simulink model "ECU_Controller"  (R2025b)
settings: Solver=FixedStepAuto  StartTime=0.0  StopTime=10.0  RelTol=1e-3  EnableMultiTasking=on
libraries: stm32f4xxblockslib x2
settings Model: STM32="{\"AnalogInput\":[{\"ID\":\"PIL_System_POTS:37\"},{\"ID\":\"PIL_System_POTS:38\"}]}"  Creator=Lakshay Taneja  LastModifiedBy=Lakshay Taneja
settings OptimizationCC: DefaultParameterBehavior=Inlined  EnhancedBackFolding=on  PassReuseOutputArgsAs=Individual arguments  ZeroExternalMemoryAtStartup=off  ZeroInternalMemoryAtStartup=off  MaxStackSize=512  OptimizeBlockOrder=speed  DifferentSizesBufferReuse=on  OptimizationCustomize=off  EfficientTunableParamExpr=on
settings DebuggingCC: ParameterTunabilityLossMsg=error
settings HardwareCC: ProdBitPerPointer=32.0  ProdBitPerSizeT=32.0  ProdBitPerPtrDiffT=32.0  ProdLargestAtomicInteger=Long  ProdLargestAtomicFloat=Double  ProdWordSize=32.0  ProdLongLongMode=on  ProdHWDeviceType=ARM Compatible->ARM Cortex-M
settings SFSimCC: MATLABDynamicMemAlloc=off
settings RTWCC: SystemTargetFile=ert.tlc  HardwareBoard=STM32F4xx Based  TemplateMakefile=ert_default_tmf  Toolchain=GNU Tools for ARM Embedded Processors  CreateSILPILBlock=PIL  Description=Embedded Coder
settings CodeAppCC: ForceParamTrailComments=on  IgnoreCustomStorageClasses=off  OperatorAnnotations=on  SimulinkDataObjDesc=on  SFDataObjDesc=on  InsertBlockDesc=on
settings ERTTargetCC: ExtModeTransport=3.0  ExtModeStaticAlloc=on  ExtModeStaticAllocSize=2048.0  ExtModeMexFile=ext_xcp  ExtModeIntrfLevel=Level2 - Open  TargetLangStandard=C99 (ISO)  CodeReplacementLibrary=ARM Cortex-M

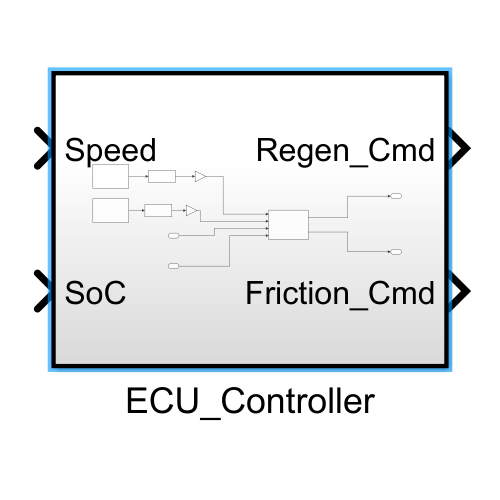
[thumbnail: Simulink's stored preview of the top-level diagram]
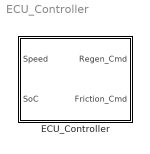
== system ECU_Controller ==
  ECU_Controller : Subsystem  TreatAsAtomicUnit=on

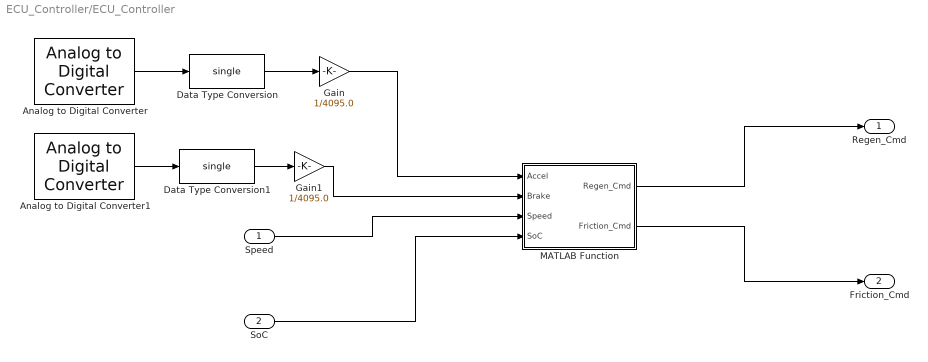
== system ECU_Controller/ECU_Controller ==
  Speed : Inport  OutDataTypeStr=single
  SoC : Inport  Port=2  OutDataTypeStr=single
  Analog to Digital Converter : stm32f4xxblockslib/Analog to Digital Converter  ADCModule=ADC1  ConversionGroup=Regular  TriggerMode=Trigger and read  NumberOfConversions=1  EnableBufferConv=off  BufferLength=1  OutputStatus=off  SampleTime=0.01  EnableSimPort=off  hoistedMaskSrc=ECSoC/ECSimCodegen/Analog to Digital Converter
      settings: LibrarySourceBlock=stm32f1xxblockslib/Analog to Digital Converter
  Analog to Digital Converter1 : stm32f4xxblockslib/Analog to Digital Converter  ADCModule=ADC2  ConversionGroup=Regular  TriggerMode=Trigger and read  NumberOfConversions=1  EnableBufferConv=off  BufferLength=1  OutputStatus=off  SampleTime=0.01  EnableSimPort=off  hoistedMaskSrc=ECSoC/ECSimCodegen/Analog to Digital Converter
      settings: LibrarySourceBlock=stm32f1xxblockslib/Analog to Digital Converter
  Data Type Conversion : DataTypeConversion  OutDataTypeStr=single  SaturateOnIntegerOverflow=off  RndMeth=Floor
  Data Type Conversion1 : DataTypeConversion  OutDataTypeStr=single  SaturateOnIntegerOverflow=off  RndMeth=Floor
  Gain : Gain  Gain=1/4095.0  OutDataTypeStr=single
  Gain1 : Gain  Gain=1/4095.0  OutDataTypeStr=single
  MATLAB Function : MATLAB Function  TreatAsAtomicUnit=on
  Regen_Cmd : Outport  OutDataTypeStr=single
  Friction_Cmd : Outport  Port=2  OutDataTypeStr=single
  wires:
  Speed/1 -> MATLAB Function/3(Speed)
  MATLAB Function/2(Friction_Cmd) -> Friction_Cmd/1
  MATLAB Function/1(Regen_Cmd) -> Regen_Cmd/1
  SoC/1 -> MATLAB Function/4(SoC)
  Analog to Digital Converter/1 -> Data Type Conversion/1
  Analog to Digital Converter1/1 -> Data Type Conversion1/1
  Gain/1 -> MATLAB Function/1(Accel)
  Gain1/1 -> MATLAB Function/2(Brake)
  Data Type Conversion/1 -> Gain/1
  Data Type Conversion1/1 -> Gain1/1

== matlab function ECU_Controller/MATLAB Function ==
  data: Accel input; Regen_Cmd output; Brake input; Speed input; SoC input; Friction_Cmd output
function [Regen_Cmd, Friction_Cmd] = ECU_Logic(Accel, Brake, Speed, SoC)
% ECU_Logic - Final Production Version
% Implements robust Torque Splitting, Safe Interpolation, and SoC Protection.
%
% Inputs:
%   Accel : Accelerator Pedal (0.0 to 1.0)
%   Brake : Brake Pedal (0.0 to 1.0)
%   Speed : Vehicle Speed (m/s) [Auto-detects km/h and converts]
%   SoC   : Battery State of Charge (0.0 to 1.0)
%
% Outputs:
%   Regen_Cmd    : Torque command for Motor (Negative = Regen) [Nm]
%   Friction_Cmd : Torque command for Friction Brakes [Nm]

%% --- 0. INITIALIZATION & SAFE CASTS ---
Regen_Cmd    = single(0);
Friction_Cmd = single(0);

% Clamp inputs to safe 0-1 range
ac_in = single(min(max(Accel, 0.0), 1.0));
br_in = single(min(max(Brake, 0.0), 1.0));
sc_in = single(min(max(SoC, 0.0), 1.0));
sp_in = single(Speed);

%% --- 1. TUNABLE PARAMETERS ---
% Torque Limits
Max_Prop_Trq    = single(2800);    % Nm (Propulsion)
Max_Brake_Trq   = single(-4500);   % Nm (Emergency Braking Limit)
One_Pedal_Trq   = single(-300);    % Nm (Coasting Drag)

% Control Thresholds
Deadband        = single(0.05);    % 5% Pedal Deadband
Zero            = single(0);
Top_Speed_Limit = single(45.0);    % m/s (approx 162 km/h)

% SoC Safety Hysteresis (Protection)
SoC_Disable_High = single(0.95);   % Cut regen above 95%
SoC_Enable_Low   = single(0.93);   % Re-enable below 93%

% Max Regen Limits for Safety Clamps
% (Used later in final check)
Limit_Min_Trq   = single(-2500); 

%% --- 2. UNIT CONVERSION PROTECTION ---
% If input speed is physically impossible for m/s (> 54 m/s), assume km/h
if sp_in > (Top_Speed_Limit * single(1.2))
    sp_in = sp_in / single(3.6);
end
sp_in = max(Zero, sp_in); % Ensure non-negative

%% --- 3. DRIVER INTENT LOGIC ---
% Priority: Brake > Accelerator > Coasting

if br_in > Deadband
    % Case: Braking
    req_prop    = Zero;
    is_coasting = false;
    
    % Linear mapping for Friction Brake Request
    req_brake = br_in * Max_Brake_Trq;
    
else
    % Case: Not Braking
    req_brake = Zero;
    
    if ac_in > Deadband && sp_in < Top_Speed_Limit
        % Case: Propulsion
        is_coasting = false;
        req_prop = ac_in * Max_Prop_Trq;
        
        % Soft Governor: Fade out torque in last 5 m/s before top speed
        if sp_in > (Top_Speed_Limit - single(5.0))
            factor = (Top_Speed_Limit - sp_in) / single(5.0);
            req_prop = req_prop * factor;
        end
    else
        % Case: Coasting (Accelerator released)
        is_coasting = true;
        req_prop = Zero;
    end
end

% One-Pedal Logic (Active only during coasting)
if is_coasting
    req_oneped = One_Pedal_Trq; % Apply -300 Nm drag
else
    req_oneped = Zero;
end

% Calculate Total Driver Demand (Nm)
total_req = req_prop + req_oneped + req_brake;

%% --- 4. REGEN ENVELOPE (EXPLICIT LOGIC) ---
% No loops. Hard-coded segments with explicit single-precision math.
% This fixes the -2500 flatline bug and the "double type" error.

max_regen_lim = Zero;

if sp_in <= single(5.0)
    % Segment 1: 0 to 5 m/s (Ramp down)
    % Slope = -200
    max_regen_lim = single(0) + (single(-200.0) * sp_in);
    
elseif sp_in <= single(10.0)
    % Segment 2: 5 to 10 m/s (Ramp down)
    % Slope = -300
    max_regen_lim = single(-1000.0) + (single(-300.0) * (sp_in - single(5.0)));
    
elseif sp_in <= single(25.0)
    % Segment 3: 10 to 25 m/s (Flat Max Torque)
    max_regen_lim = single(-2500.0);
    
elseif sp_in <= single(45.0)
    % Segment 4: 25 to 45 m/s (Field Weakening Ramp Up)
    % Slope = 65
    max_regen_lim = single(-2500.0) + (single(65.0) * (sp_in - single(25.0)));
    
else 
    % Above 45 m/s (Safety clamp)
    max_regen_lim = single(-1200.0);
end

% Final Safety Clamp (Ensure strictly negative or zero)
max_regen_lim = min(Zero, max_regen_lim);

%% --- 5. BATTERY PROTECTION (SoC HYSTERESIS) ---
% State Machine to prevent rapid toggling near 95% SoC
persistent regen_disabled
if isempty(regen_disabled)
    regen_disabled = false;
end

if ~regen_disabled
    if sc_in > SoC_Disable_High
        regen_disabled = true; % Cutoff
    end
else
    if sc_in < SoC_Enable_Low
        regen_disabled = false; % Reset
    end
end

% Determine final available regen capability
if regen_disabled
    avail_regen = Zero;
else
    avail_regen = max_regen_lim;
end

%% --- 6. TORQUE SPLIT ALGORITHM ---
% Arbitrates between Motor and Friction Brakes

if total_req >= Zero
    % A. PROPULSION
    % Motor handles everything. Friction is zero.
    calc_regen = min(total_req, Max_Prop_Trq);
    calc_frict = Zero;
    
else
    % B. BRAKING
    % 1. Maximize Regen first (limited by avail_regen curve)
    %    Note: Since both are negative, max() selects the one closer to 0.
    %    Ex: max(-2000 req, -2500 lim) -> -2000 (Full Regen)
    %    Ex: max(-4000 req, -2500 lim) -> -2500 (Regen Saturated)
    calc_regen = max(total_req, avail_regen);
    
    % 2. Friction fills the gap
    %    Friction = Total - Regen
    calc_frict = total_req - calc_regen;
end

%% --- 7. FINAL SAFETY CLAMPS ---
% Ensure Motor command is within physical limits
calc_regen = max(calc_regen, Limit_Min_Trq); % Can't be more neg than -2500
calc_regen = min(calc_regen, Max_Prop_Trq);

% Ensure Friction command is strictly negative (braking only)
calc_frict = min(calc_frict, Zero);
calc_frict = max(calc_frict, Max_Brake_Trq);

%% --- 8. OUTPUT ASSIGNMENT ---
Regen_Cmd    = single(calc_regen);
Friction_Cmd = single(calc_frict);

end
